simulink model "ADU_Integration_Y2016_simulation"  (R2016b)
settings: Solver=FixedStepDiscrete  StartTime=240  StopTime=300  FixedStep=0.01  RelTol=1e-3  EnableMultiTasking=on
PostLoadFcn:
  | , if any(exist('dsrtsu_mdlpostloadfcn', 'file') == [2, 3, 6]), try dsrtsu_mdlpostloadfcn('Execute', bdroot); catch fprintf('Error in PostLoadFcn (dsrtsu_mdlpostloadfcn) for model "%s":\n %s\n', bdroot, lasterr); end, end,
InitFcn:
  | load 'data/chi2_dat';
  | load 'data/innerLine_struct';
  | load 'data/middleLine_struct';
  | load 'data/outerLine_struct';
  | load 'data/innerLine';
  | load 'data/middleLine';
  | load 'data/outerLine';
  | load 'data/landmarks_patac_schimmel_ccw';
  | load 'data/patac_navi_array';
  | load 'data/sensor';
  | load 'data/map_struct';
  | addpath map_src
  | Integration_Parameter;
  | load 'TestData_001';
values from neighbouring files (symbols this model uses):
  TestData_001 =     [TestData_001.mat]
undefined symbols (not defined in the file or in its folder): chi2_dat, innerLine, landmarks_patac_schimmel_ccw, middleLine, outerLine, patac_navi_array
libraries: simulink x36, rtican x1
(part 1 of 20)
settings Model: DSRTSU_INTERNAL_RTI_VER=460  DSRTSU_INTERNAL_RTI_TYPE=rti1401  DSRTSU_INTERNAL_RTIFLEXRAYCONFIG=10  DSRTSU_INTERNAL_RTIFPGA=50  Creator=si8cwy  LastModifiedBy=Administrator
settings DataIOCC: LimitDataPoints=on  SaveFormat=Array  SignalLoggingSaveFormat=ModelDataLogs
settings OptimizationCC: BlockReduction=off  ConditionallyExecuteInputs=off  OptimizeBlockIOStorage=off  BufferReuse=off  GlobalBufferReuse=off  ExpressionFolding=off  ExpressionDepthLimit=2147483647  LocalBlockOutputs=off  RollThreshold=100  LifeSpan=inf
settings DebuggingCC: SolverPrmCheckMsg=warning  MultiTaskDSMMsg=warning  MultiTaskCondExecSysMsg=none  StateNameClashWarn=warning  SFUnexpectedBacktrackingDiag=warning  SFNoUnconditionalDefaultTransitionDiag=warning  SFExecutionAtInitializationDiag=none
settings HardwareCC: ProdBitPerPointer=32  ProdBitPerSizeT=32  ProdBitPerPtrDiffT=32  ProdLargestAtomicFloat=None  ProdEndianess=BigEndian  ProdWordSize=32  ProdHWDeviceType=Generic->Custom  TargetIntDivRoundTo=Zero  TargetEndianess=BigEndian  TargetHWDeviceType=Generic->Custom
settings ModelReferenceCC: PropagateSignalLabelsOutOfModel=off
settings RTWCC: SystemTargetFile=rti1401.tlc  MakeCommand=make_rti  TemplateMakefile=rti1401.tmf  Description=dSPACE DS1401 Hardware Platform
settings STFCustomTargetCC: ParMdlRefBuildCompliant=on  SystemTargetFile=rti1401.tlc
settings GRTTargetCC: TargetLangStandard=C89/C90 (ANSI)  CompOptLevelCompliant=off  ConcurrentExecutionCompliant=off  CombineOutputUpdateFcns=off  MatFileLogging=off  CPPClassGenCompliant=off  GRTInterface=on  UseToolchainInfoCompliant=off  ExtModeMexFile=noextcomm
settings ConfigComp: CovMetricSettings=dw  CovHtmlReporting=on  CovSaveCumulativeToWorkspaceVar=on  CovSaveSingleToWorkspaceVar=on  CovExternalEMLEnable=off  CovSFcnEnable=off

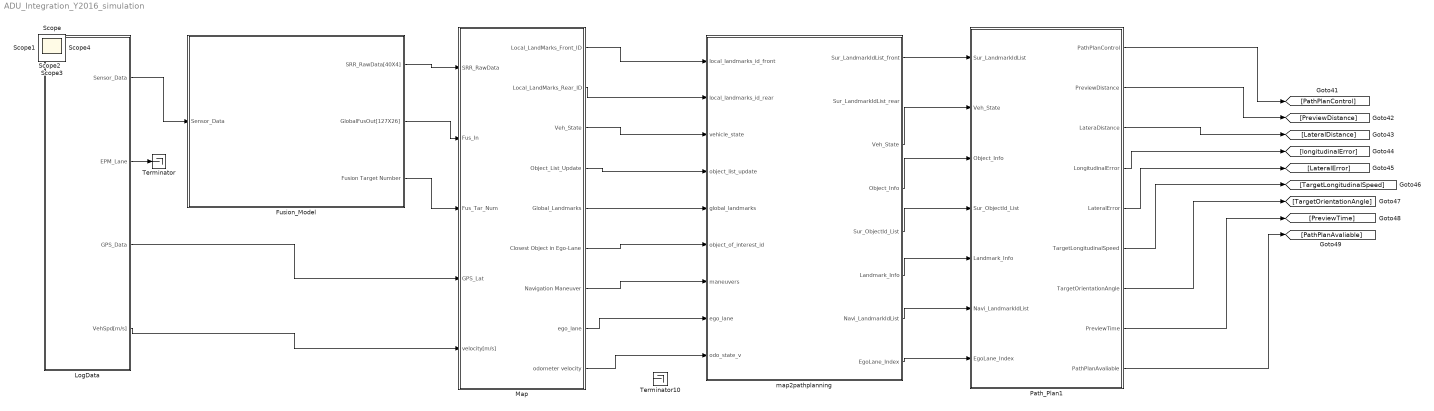
== system ADU_Integration_Y2016_simulation ==
  Fusion_Model : Subsystem
  LogData : Subsystem
  Map : Subsystem
  Path_Plan1 : Subsystem
  Terminator : Terminator
  Terminator10 : Terminator
  map2pathplanning : MATLAB Function  TreatAsAtomicUnit=on
  Scope{,1..4} (5 alike) : Scope
  wires:
  LogData/1(Sensor_Data) -> Fusion_Model/1(Sensor_Data)
  LogData/2(EPM_Lane) -> Terminator/1
  Path_Plan1/1(PathPlanControl) -> [PathPlanControl]
  Path_Plan1/2(PreviewDistance) -> [PreviewDistance]
  Path_Plan1/3(LateraDistance) -> [LateralDistance]
  Path_Plan1/9(PathPlanAvaliable) -> [PathPlanAvaliable]
  Path_Plan1/8(PreviewTime) -> [PreviewTime]
  Path_Plan1/4(LongitudinalError) -> [longitudinalError]
  Path_Plan1/5(LateralError) -> [LateralError]
  Path_Plan1/7(TargetOrientationAngle) -> [TargetOrientationAngle]
  Path_Plan1/6(TargetLongitudinalSpeed) -> [TargetLongitudinalSpeed]
  map2pathplanning/8(EgoLane_Index) -> Path_Plan1/7(EgoLane_Index)
  map2pathplanning/7(Navi_LandmarkIdList) -> Path_Plan1/6(Navi_LandmarkIdList)
  map2pathplanning/5(Sur_ObjectId_List) -> Path_Plan1/4(Sur_ObjectId_List)
  map2pathplanning/3(Veh_State) -> Path_Plan1/2(Veh_State)
  map2pathplanning/4(Object_Info) -> Path_Plan1/3(Object_Info)
  map2pathplanning/1(Sur_LandmarkIdList_front) -> Path_Plan1/1(Sur_LandmarkIdList)
  map2pathplanning/6(Landmark_Info) -> Path_Plan1/5(Landmark_Info)
  Map/1(Local_LandMarks_Front_ID) -> map2pathplanning/1(local_landmarks_id_front)
  Map/3(Veh_State) -> map2pathplanning/3(vehicle_state)
  Map/4(Object_List_Update) -> map2pathplanning/4(object_list_update)
  Map/5("Global_Landmarks ") -> map2pathplanning/5(global_landmarks)
  Map/6(Closest Object in Ego-Lane) -> map2pathplanning/6(object_of_interest_id)
  Map/7(Navigation Maneuver) -> map2pathplanning/7(maneuvers)
  Map/9(odometer velocity) -> map2pathplanning/9(odo_state_v)
  Map/8(ego_lane) -> map2pathplanning/8(ego_lane)
  Fusion_Model/2(GlobalFusOut[127X26]) -> Map/2(Fus_In)
  Fusion_Model/1(SRR_RawData[40X4]) -> Map/1(SRR_RawData)
  LogData/3(GPS_Data) -> Map/4(GPS_Lat)
  LogData/4(VehSpd[m/s]) -> Map/5(velocity[m/s])
  Map/2(Local_LandMarks_Rear_ID) -> map2pathplanning/2(local_landmarks_id_rear)
  Fusion_Model/3(Fusion Target Number) -> Map/3(Fus_Tar_Num)

== system ADU_Integration_Y2016_simulation/Fusion_Model ==
  note: SRR  Data
      | --------------------------------------------------------
      | |  1  |     2       |      3       |       4       |
      | --------------------------------------------------------
      | | ID | RangeX | RangeY | MoveInfo |
  note: Model Description:
      | This Model now don't take SRR Data to initial fusion tracker, the side fusion strategy will develop and update the model,
      | all output is based on vehicle coordinate, which original point located on the front middle of vehicle, the vehicle is 1.8m
      | wide and 5.2m long. Now the Move Info signal and Fus_State is unavialbe, The fusion output has two way, the 127x26
      | and 127 object is optional,the EPM Obstacle is used for ACC Strategy, not used for path plan and motion control.
  note: FusDataOut  Data
      | ------------------------------------------------------------------------------------------------------------------------------------------------------------------------------------------------------------------------------------------------------------------------------------------------------
      | |  1  |     2       |   3    |     4        |    5   |        6       |   7      |   8    |        9        |         10      |   11  |  12  |  13  |  14   | 15   |  16  |  17   |  18  |  19  |   20  |  21  |  22  |   23  |  24  |  25  |  26   |
      | -----------------------------------------------------------------------------------------------------------------------------------------------------------------------------------------------------------------------------------------------------------------------------------------------------
      | | ID | RangeX | VelX | RangeY | VelY | MoveInfo | Width | Type | Fus_State | Confidence| P11 | P12 | P13 | P14 | P21 | P22 | P23 | P24 | P31 | P32 | P33 | P34 | P41 | P42 | P43 | P44 |
  Sensor_Data : Inport
  DocBlock : simulink/Model-Wide Utilities/DocBlock  DocumentType=Text
      content=|
      | V1.0
      | 2016/11/1   |   First Release
      | V2.0
      | 2016/11/7   |   Changelog:
      | 1)  Output all SRR Raw Data, used for map;
      | 2)  Updating EPM dbc, new feature is avaliable;
      | 3)  Add Obstacle_State A/B/C for acc control;
      | 4)  Add FreeSpace and HPP signal for other use.
  Fusion_Block : Subsystem
  To Workspace : ToWorkspace  VariableName=FusOut  SampleTime=-1
  SRR_RawData[40X4] : Outport
  GlobalFusOut[127X26] : Outport  Port=2
  Fusion Target Number : Outport  Port=3
  wires:
  Fusion_Block/1(Fus_Data_Out) -> To Workspace/1, GlobalFusOut[127X26]/1
  Fusion_Block/3(SRR_RawData) -> SRR_RawData[40X4]/1
  Sensor_Data/1 -> Fusion_Block/1(Sensor_Data)
  Fusion_Block/2(fusion target number) -> Fusion Target Number/1

== system ADU_Integration_Y2016_simulation/LogData ==
  1-D Lookup Table2 : Lookup_n-D  NumberOfTableDimensions=1  BreakpointsForDimension1=TestData_001.X.Data  Table=TestData_001.Y(731).Data  RndMeth=Simplest  InputSameDT=on
  Bus Creator : BusCreator  Inputs=6
  Clock : Clock
  LF_SRR_Data : Subsystem
  LR_SRR_Data : Subsystem
  RF_SRR_Data : Subsystem
  RR_SRR_Data : Subsystem
  SER_M2S : Subsystem
  Sensor_ESR : Subsystem
  Vision_Target : Subsystem
  Sensor_Data : Outport
  EPM_Lane : Outport  Port=2
  GPS_Data : Outport  Port=3
  VehSpd[m/s] : Outport  Port=4
  tag scope: Clock=global
  wires:
  LF_SRR_Data/1(LF_SRR_Data[10x5]) -> Bus Creator/2  "LF_SRR_Data[10X5]"
  RF_SRR_Data/1(RF_SRR_Data[10x5]) -> Bus Creator/3  "RF_SRR_Data[10X5]"
  LR_SRR_Data/1(LR_SRR_Data[10x5]) -> Bus Creator/4  "LR_SRR_Data[10X5]"
  RR_SRR_Data/1(RR_SRR_Data[10x5]) -> Bus Creator/5  "RR_SRR_Data[10X5]"
  Vision_Target/1(Vision_Target[25x8]) -> Bus Creator/6  "Vision_Target[25X8]"
  Bus Creator/1 -> Sensor_Data/1  "Sensor_Veh_Data"
  Sensor_ESR/1(ESR_Data[64X4]) -> Bus Creator/1  "ESR_Data[64X4]"
  Vision_Target/2(EPM_Lane) -> EPM_Lane/1
  Clock/1 -> [Clock]
  SER_M2S/1(NET_Output) -> GPS_Data/1
  [Clock] -> 1-D Lookup Table2/1
  1-D Lookup Table2/1 -> VehSpd[m/s]/1

== system ADU_Integration_Y2016_simulation/Map ==
  SRR_RawData : Inport
  Fus_In : Inport  Port=2
  Fus_Tar_Num : Inport  Port=3
  GPS_Lat : Inport  Port=4
  velocity[m/s] : Inport  Port=5
  Bus Selector2 : BusSelector  OutputSignals=GPGLL.Y_Lat,GPGLL.Y_Long,GPHPR.Crouse_Range,GPGLL.Time[s]
  Constant : Constant  Value=chi2_dat
  Constant1 : Constant  Value=middleLine  OutDataTypeStr=Bus: middleLine_struct
  Constant2 : Constant  Value=innerLine  OutDataTypeStr=Bus: innerLine_struct
  Constant3 : Constant  Value=outerLine  OutDataTypeStr=Bus: outerLine_struct
  Constant5 : Constant  Value=patac_navi_array  OutDataTypeStr=double
  Data Store Memory2 : DataStoreMemory  DataStoreName=chi2  ReadBeforeWriteMsg=warning  WriteAfterWriteMsg=warning  WriteAfterReadMsg=warning  InitialValue=zeros(1,1000)  ShowAdditionalParam=off  OutDataTypeStr=double
  Display : Display
  Map_Navigation : MATLAB Function  TreatAsAtomicUnit=on
  Terminator4 : Terminator
  landmarks_patac_schimmel_ccw : Constant  Value=landmarks_patac_schimmel_ccw  OutDataTypeStr=double
  Local_LandMarks_Front_ID : Outport
  Local_LandMarks_Rear_ID : Outport  Port=2
  Veh_State : Outport  Port=3
  Object_List_Update : Outport  Port=4
  "Global_Landmarks " : Outport  Port=5
  Closest Object in Ego-Lane : Outport  Port=6
  Navigation Maneuver : Outport  Port=7
  ego_lane : Outport  Port=8
  odometer velocity : Outport  Port=9
  wires:
  Map_Navigation/3(object_list_update) -> Object_List_Update/1
  Map_Navigation/2(vehicle_state) -> Display/1, Veh_State/1
  velocity[m/s]/1 -> Map_Navigation/6(odo_motion_v)
  GPS_Lat/1 -> Bus Selector2/1
  Bus Selector2/1 -> Map_Navigation/7(rtk_gps_lat)  "<Y_Lat>"
  Bus Selector2/2 -> Map_Navigation/8(rtk_gps_lon)  "<Y_Long>"
  Bus Selector2/3 -> Map_Navigation/9(rtk_gps_yaw)  "<Crouse_Range>"
  Bus Selector2/4 -> Map_Navigation/10(rtk_gps_ts)  "<Time[s]>"
  SRR_RawData/1 -> Map_Navigation/11(sensor_data_raw)
  Fus_In/1 -> Map_Navigation/12(object_list)
  Map_Navigation/4(object_of_interest_id) -> Closest Object in Ego-Lane/1
  Map_Navigation/7(maneuvers) -> Navigation Maneuver/1
  Constant/1 -> Map_Navigation/1(chi2_dat)
  Constant2/1 -> Map_Navigation/2(innerLine)
  Constant1/1 -> Map_Navigation/3(middleLine)
  Constant3/1 -> Map_Navigation/4(outerLine)
  landmarks_patac_schimmel_ccw/1 -> Map_Navigation/5(landmarks)
  Constant5/1 -> Map_Navigation/14(patac_navi)
  ? -> Terminator4/1
  Map_Navigation/12(odo_state_v) -> odometer velocity/1
  Map_Navigation/5(landmarks_in_proximity_id_in_front) -> Local_LandMarks_Front_ID/1
  Map_Navigation/1(global_landmarks) -> "Global_Landmarks "/1
  Map_Navigation/11(ego_location) -> ego_lane/1
  Map_Navigation/6(landmarks_in_proximity_id_in_rear) -> Local_LandMarks_Rear_ID/1
  Fus_Tar_Num/1 -> Map_Navigation/13(object_num)

== system ADU_Integration_Y2016_simulation/Path_Plan1 ==
  note: Veh_State
      | |  1 |  2  |    3   |  4  |  5  |  6  |  7  | 8 |
      | -------------------------------------------------
      | | X  | Y  | Beta | Vx | Vy | Ax | Ay | V |
  note: FusDataOut  Data
      | ------------------------------------------------------------------------------------------------------------------------------------------------------------------------------------------------------------------------------------------------------
      | |  1  |     2       |   3    |     4        |    5   |        6       |   7      |   8    |        9        |         10      |   11  |  12  |  13  |  14   | 15   |  16  |  17   |  18  |  19  |   20  |  21  |  22  |   23  |  24  |  25  |  26   |
      | -------------------------------------------------------------------------------------------------------------------------------------------------------------------------------------------------------------------------------------------------------
      | | ID | RangeX | VelX | RangeY | VelY | MoveInfo | Width | Type | Fus_State | Confidence| P11 | P12 | P13 | P14 | P21 | P22 | P23 | P24 | P31 | P32 | P33 | P34 | P41 | P42 | P43 | P44 |
  note: Landmark_Info
      | |   1  |   2   |   3   |   4  |    5    |
      | ---------------------------------------- X 30
      | | X1  | Y1  |  X2  |  Y2 | Type |
  note: Sur_LandmarkIdList
      | |  1  |  2  |  3  |  4  |  5  |  6  |  7  |  8  |  9  |  10  |
      | --------------------------------------------------------------
      | | id  |
  note: Navi_LandmarkIdList
      | |  1  |  2  |      3      |    4   |
      | ----------------------------------
      | |  x  |  y  |  Range  |  OP  |
  note: Sur_ObjectId_List
      | |  1  |  2  |  3  |  4  |
      | -------------------------  1stLane   2ndLane  3rdLane
      | | id  |
  Sur_LandmarkIdList : Inport
  Veh_State : Inport  Port=2
  Object_Info : Inport  Port=3
  Sur_ObjectId_List : Inport  Port=4
  Landmark_Info : Inport  Port=5
  Navi_LandmarkIdList : Inport  Port=6
  EgoLane_Index : Inport  Port=7
  Constant : Constant
  CordTransfer : MATLAB Function  TreatAsAtomicUnit=on
  CordTransfer1 : MATLAB Function  TreatAsAtomicUnit=on
  Demux : Demux
  Demux1 : Demux
  Demux2 : Demux  Outputs=8
  InterSectionPathPlanningModule : Subsystem
  LaneChangePathPlanningModule1 : Subsystem
  PathArbModule : Subsystem
  SceneSelectionModule : Subsystem
  Terminator : Terminator
  Terminator1 : Terminator
  Terminator2 : Terminator
  Unit Delay : UnitDelay  InitialCondition=1  SampleTime=-1
  PathPlanControl : Outport
  PreviewDistance : Outport  Port=2
  LateraDistance : Outport  Port=3
  LongitudinalError : Outport  Port=4
  LateralError : Outport  Port=5
  TargetLongitudinalSpeed : Outport  Port=6
  TargetOrientationAngle : Outport  Port=7
  PreviewTime : Outport  Port=8
  PathPlanAvaliable : Outport  Port=9
  wires:
  Unit Delay/1 -> SceneSelectionModule/8(OperationFinishFlg)
  PathArbModule/6(PathTrigFinishFlg) -> Unit Delay/1
  LaneChangePathPlanningModule1/6(PathTrigFinishFlg) -> PathArbModule/12(PathTrigFinishFlgLC)
  InterSectionPathPlanningModule/6(PathTrigFinishFlg) -> PathArbModule/6(PathTrigFinishFlgInter)
  LaneChangePathPlanningModule1/5(PreViewTime) -> PathArbModule/11(PreviewTimeLC)
  LaneChangePathPlanningModule1/4(TargetThetalo) -> PathArbModule/10(TargetThetaLoLC)
  LaneChangePathPlanningModule1/3(PathPlanningSuccessFlg) -> PathArbModule/9(VePathPlan_e_LCPPSucFlg)
  LaneChangePathPlanningModule1/2(VsPathPlan_h_Motion) -> PathArbModule/8(VsPathPlan_h_LCMotion)
  LaneChangePathPlanningModule1/1(VsPathPlan_h_position) -> PathArbModule/7(VsPathPlan_h_LCposition)
  InterSectionPathPlanningModule/5(PreViewTime) -> PathArbModule/5(PreviewTimeInter)
  InterSectionPathPlanningModule/4(TargetThetalo) -> PathArbModule/4(TargetThetaLoInter)
  InterSectionPathPlanningModule/3(PathPlanningSuccessFlg) -> PathArbModule/3(VePathPlan_e_InterPPSucFlg)
  InterSectionPathPlanningModule/2(VsPathPlan_h_Motion) -> PathArbModule/2(VsPathPlan_h_InterSecMotion)
  InterSectionPathPlanningModule/1(VsPathPlan_h_position) -> PathArbModule/1(VsPathPlan_h_InterSecposition)
  PathArbModule/3(VePathPlan_b_InChargFlg) -> PathPlanControl/1
  PathArbModule/2(VsPathPlan_h_Motion) -> Demux1/1, CordTransfer1/3(VsPathPlan_h_MotionPGC)
  PathArbModule/1(VsPathPlan_h_position) -> Demux/1, CordTransfer1/2(VsPathPlan_h_positionPGC)
  PathArbModule/5(PreviewTime) -> PreviewTime/1
  PathArbModule/4(TargetThetaLo) -> TargetOrientationAngle/1, CordTransfer1/4(TargetThetaLoPGC)
  Demux1/1 -> TargetLongitudinalSpeed/1
  Demux/4 -> LateralError/1
  Demux/3 -> LongitudinalError/1
  Demux/2 -> LateraDistance/1
  Demux/1 -> PreviewDistance/1
  Constant/1 -> PathPlanAvaliable/1
  CordTransfer/6(Info_LoPGCd) -> LaneChangePathPlanningModule1/10(Info_Lo)
  CordTransfer/5(Info_LdPGCd) -> InterSectionPathPlanningModule/4(Info_Ld), LaneChangePathPlanningModule1/9(Info_Ld)
  CordTransfer/3(Info_FdPGCd) -> InterSectionPathPlanningModule/5(Info_Fd), LaneChangePathPlanningModule1/7(Info_Fd)
  Demux2/2 -> InterSectionPathPlanningModule/7(YposLoCur), LaneChangePathPlanningModule1/3(YposLoCur)
  Demux2/3 -> InterSectionPathPlanningModule/8(ThetaLoCur), LaneChangePathPlanningModule1/4(ThetaLoCur)
  CordTransfer/4(Info_FoPGCd) -> LaneChangePathPlanningModule1/8(Info_Fo)
  CordTransfer/1(Info_MePGCd) -> InterSectionPathPlanningModule/1(Info_Me), LaneChangePathPlanningModule1/1(Info_Me)
  Demux2/1 -> InterSectionPathPlanningModule/6(XposLoCur), LaneChangePathPlanningModule1/2(XposLoCur)
  CordTransfer/8(CurOpPGCd) -> InterSectionPathPlanningModule/3(VePathPlanning_e_CurOp), LaneChangePathPlanningModule1/6(VePathPlanning_e_CurOp), PathArbModule/13(VePathPlan_e_OutputSelection)
  Sur_LandmarkIdList/1 -> SceneSelectionModule/1(Sur_LandmarkIdList)
  Veh_State/1 -> Demux2/1, SceneSelectionModule/2(Veh_State)
  Navi_LandmarkIdList/1 -> SceneSelectionModule/6(Navi_LandmarkIdList)
  Landmark_Info/1 -> SceneSelectionModule/5(Landmark_Info)
  Sur_ObjectId_List/1 -> SceneSelectionModule/4(Sur_ObjectId_List)
  Object_Info/1 -> SceneSelectionModule/3(Object_Info)
  EgoLane_Index/1 -> SceneSelectionModule/7(EgoLane_Index)
  CordTransfer/2(RoadInfoPGCd) -> InterSectionPathPlanningModule/2(RoadInfo), LaneChangePathPlanningModule1/5(RoadInfo)
  CordTransfer/7(LongDisLimitPGCd) -> LaneChangePathPlanningModule1/11(LongDisLimit)
  SceneSelectionModule/1(Info_Me) -> CordTransfer/1(Info_MeGCd)
  SceneSelectionModule/2(Info_Fd) -> CordTransfer/2(Info_FdGCd)
  SceneSelectionModule/3(Info_Fo) -> CordTransfer/3(Info_FoGCd)
  SceneSelectionModule/5(Info_Lo) -> CordTransfer/5(Info_LoGCd)
  SceneSelectionModule/6(CurOp) -> CordTransfer/6(CurOpGCd)
  SceneSelectionModule/4(Info_Ld) -> CordTransfer/4(Info_LdGCd)
  SceneSelectionModule/7(LongDisLimit) -> CordTransfer/7(LongDisLimitGCd)
  SceneSelectionModule/8(RoadInfo) -> CordTransfer/8(RoadInfoGCd)
  CordTransfer/9(PGCdInfo) -> CordTransfer1/1(PGCdInfo)
  CordTransfer1/3(TargetThetaLo) -> Terminator2/1
  CordTransfer1/2(VsPathPlan_h_Motion) -> Terminator1/1
  CordTransfer1/1(VsPathPlan_h_position) -> Terminator/1

== system ADU_Integration_Y2016_simulation/Fusion_Model/Fusion_Block ==
  Sensor_Data : Inport
  Bus Selector : BusSelector  OutputSignals=Total_Targ_Num
  Display : Display
  Fus_Header_Gen : Subsystem
  Global_Fusion : Subsystem
  Side_Fusion : Subsystem
  Terminator : Terminator
  Fus_Data_Out : Outport
  fusion target number : Outport  Port=2
  SRR_RawData : Outport  Port=3
  wires:
  Side_Fusion/1(SideFus_Output[40X4]) -> Global_Fusion/1(From SideFusion)
  Global_Fusion/1(GlobalFusOut[127X26]) -> Fus_Data_Out/1
  Sensor_Data/1 -> Side_Fusion/1(From Sensor), Global_Fusion/2(From Sensor)
  Global_Fusion/2(Total_TargetNum) -> Display/1, Fus_Header_Gen/1(Target_Num)
  Side_Fusion/2(SideRadar_RawData[40X4]) -> SRR_RawData/1
  Fus_Header_Gen/1(Fus_Header) -> Bus Selector/1, Terminator/1
  Bus Selector/1 -> fusion target number/1  "<Total_Targ_Num>"

== system ADU_Integration_Y2016_simulation/LogData/LF_SRR_Data ==
  note: This part is used for ensure the sensor data is from once update
  1-D Lookup Table : Lookup_n-D  NumberOfTableDimensions=1  BreakpointsForDimension1=TestData_001.X.Data  Table=TestData_001.Y(51).Data  RndMeth=Simplest  InputSameDT=on
  Chart : Stateflow chart  TreatAsAtomicUnit=on
  LFSRR_Data : Subsystem
  LF_SRR_Data[10x5] : Outport
  tag scope: LFSRRTime=global, LFSRRcal=global
  wires:
  LFSRR_Data/1(LFSRR[10X5]) -> Chart/2(DataInput)
  1-D Lookup Table/1 -> Chart/1(Trig), [LFSRRcal]
  Chart/1(DataOutput) -> LF_SRR_Data[10x5]/1
  [Clock] -> Chart/3(Time), 1-D Lookup Table/1
  Chart/2(Time_out) -> [LFSRRTime]

== system ADU_Integration_Y2016_simulation/LogData/LR_SRR_Data ==
  1-D Lookup Table : Lookup_n-D  NumberOfTableDimensions=1  BreakpointsForDimension1=TestData_001.X.Data  Table=TestData_001.Y(51*2).Data  RndMeth=Simplest  InputSameDT=on
  Chart : Stateflow chart  TreatAsAtomicUnit=on
  LRSRR_Data : Subsystem  mask{StartNum=52}
  Rate Transition3 : RateTransition  Deterministic=off
  LR_SRR_Data[10x5] : Outport
  tag scope: LRSRRTime=global, LRSRRcal=global
  wires:
  Chart/1(DataOutput) -> Rate Transition3/1
  1-D Lookup Table/1 -> Chart/1(Trig), [LRSRRcal]
  Rate Transition3/1 -> LR_SRR_Data[10x5]/1
  [Clock] -> Chart/3(Time), 1-D Lookup Table/1
  LRSRR_Data/1(LRSRR[10X5]) -> Chart/2(DataInput)
  Chart/2(Time_out) -> [LRSRRTime]

== system ADU_Integration_Y2016_simulation/LogData/RF_SRR_Data ==
  1-D Lookup Table : Lookup_n-D  NumberOfTableDimensions=1  BreakpointsForDimension1=TestData_001.X.Data  Table=TestData_001.Y(153).Data  RndMeth=Simplest  InputSameDT=on
  Chart : Stateflow chart  TreatAsAtomicUnit=on
  RFSRR_Data : Subsystem  mask{StartNum=103}
  RF_SRR_Data[10x5] : Outport
  tag scope: RFSRRTime=global, RFSRRcal=global
  wires:
  1-D Lookup Table/1 -> Chart/1(Trig), [RFSRRcal]
  Chart/1(DataOutput) -> RF_SRR_Data[10x5]/1
  [Clock] -> Chart/3(Time), 1-D Lookup Table/1
  RFSRR_Data/1(RFSRR[10X5]) -> Chart/2(DataInput)
  Chart/2(Time_out) -> [RFSRRTime]

== system ADU_Integration_Y2016_simulation/LogData/RR_SRR_Data ==
  1-D Lookup Table : Lookup_n-D  NumberOfTableDimensions=1  BreakpointsForDimension1=TestData_001.X.Data  Table=TestData_001.Y(51*4).Data  RndMeth=Simplest  InputSameDT=on
  Chart : Stateflow chart  TreatAsAtomicUnit=on
  LRSRR_Data : Subsystem  mask{StartNum=154}
  RR_SRR_Data[10x5] : Outport
  tag scope: RRSRRTime=global, RRSRRcal=global
  wires:
  LRSRR_Data/1(RRSRR[10X5]) -> Chart/2(DataInput)
  [Clock] -> Chart/3(Time), 1-D Lookup Table/1
  1-D Lookup Table/1 -> Chart/1(Trig), [RRSRRcal]
  Chart/1(DataOutput) -> RR_SRR_Data[10x5]/1
  Chart/2(Time_out) -> [RRSRRTime]

== system ADU_Integration_Y2016_simulation/LogData/SER_M2S ==
  1-D Lookup Table1 : Lookup_n-D  NumberOfTableDimensions=1  BreakpointsForDimension1=TestData_001.X.Data  Table=TestData_001.Y(739).Data  RndMeth=Simplest  InputSameDT=on
  1-D Lookup Table2 : Lookup_n-D  NumberOfTableDimensions=1  BreakpointsForDimension1=TestData_001.X.Data  Table=TestData_001.Y(738).Data  RndMeth=Simplest  InputSameDT=on
  1-D Lookup Table3 : Lookup_n-D  NumberOfTableDimensions=1  BreakpointsForDimension1=TestData_001.X.Data  Table=TestData_001.Y(740).Data  RndMeth=Simplest  InputSameDT=on
  1-D Lookup Table4 : Lookup_n-D  NumberOfTableDimensions=1  BreakpointsForDimension1=TestData_001.X.Data  Table=TestData_001.Y(740).Data  RndMeth=Simplest  InputSameDT=on
  1-D Lookup Table5 : Lookup_n-D  NumberOfTableDimensions=1  BreakpointsForDimension1=TestData_001.X.Data  Table=TestData_001.Y(734).Data  RndMeth=Simplest  InputSameDT=on
  1-D Lookup Table6 : Lookup_n-D  NumberOfTableDimensions=1  BreakpointsForDimension1=TestData_001.X.Data  Table=TestData_001.Y(735).Data  RndMeth=Simplest  InputSameDT=on
  1-D Lookup Table7 : Lookup_n-D  NumberOfTableDimensions=1  BreakpointsForDimension1=TestData_001.X.Data  Table=TestData_001.Y(736).Data  RndMeth=Simplest  InputSameDT=on
  Bus Creator : BusCreator  Inputs=3
  Bus Creator1 : BusCreator  Inputs=4
  Bus Creator2 : BusCreator  Inputs=2
  NET_Output : Outport
  wires:
  1-D Lookup Table3/1 -> Bus Creator/3  "Time[s]"
  1-D Lookup Table2/1 -> Bus Creator/1  "Y_Lat"
  1-D Lookup Table1/1 -> Bus Creator/2  "Y_Long"
  Bus Creator2/1 -> NET_Output/1
  Bus Creator1/1 -> Bus Creator2/2  "GPHPR"
  1-D Lookup Table6/1 -> Bus Creator1/3  "Pitch_angle"
  1-D Lookup Table5/1 -> Bus Creator1/2  "Crouse_Range"
  Bus Creator/1 -> Bus Creator2/1  "GPGLL"
  1-D Lookup Table4/1 -> Bus Creator1/1  "Time"
  1-D Lookup Table7/1 -> Bus Creator1/4  "Roll_angle"
  [Clock] -> 1-D Lookup Table2/1, 1-D Lookup Table1/1, 1-D Lookup Table7/1, 1-D Lookup Table6/1, 1-D Lookup Table5/1, 1-D Lookup Table4/1, 1-D Lookup Table3/1

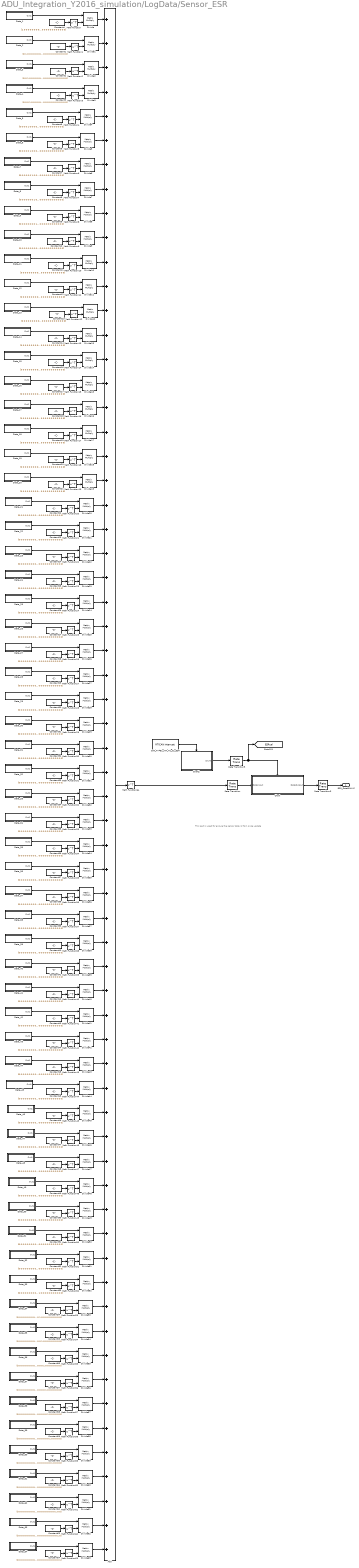
== system ADU_Integration_Y2016_simulation/LogData/Sensor_ESR ==
  note: This part is used for ensure the sensor data is from once update
  Add : Sum  Inputs=++++++++++++++++++++++++++++++++++++++++++++++++++++++++++++++++
  CAN_TYPE1_INT_M1_C1_ESR : rtican/RTICAN Interrupt  Reserved1=[]  Reserved2=[]  Reserved3=[]  Reserved4=[]  BoardTypeNo=[]  BoardNo=[]  ChannelNo=[]  Parameters=[]  InterruptName=[]  BoardIntNo=[]  Sfcn_Int_Struct=[]  BoardType=[]  SintNo=[]  Int_Struct=[]  DialogFcn=[]  UnitName=[]  Revision=[]  UnitValues=[]  DSProperties=struct('RTI',struct('Version',uint32(4),'BlockType',struct('isSLSource',uint8(1),'isSLSink',uint8(0),'isHWSource',uint8(1),'isHWSink',uint8(0),'isSetup',uint8(0),'isInline',uint8(1),'isNonInline',uint8(0),'isInterrupt',uint8(1),'isChannelwise',uint8(0)),'IOBoardType','RTICAN','UnitType','HWINT','Identifier','CANINT','DialogType','ML','BlockSet','RTICAN','RelationId',struct('TH',struct('BlockId','HWINT')),'SlaveProcessor','CAN'))  RTIBlockInterface=struct('OutputPortsWidth',int32(1),'FunctionCall',uint32(0),'OutputPortsActive',1,'DialogFcn','rtican_interrupt_gui','BlockDisplay',{{['CAN RX Interrupt'],'center'}},'IconTransparency','off','ParameterTunableNames',{{}},'InitLevel',3,'BlockName',struct('Token',{{'CAN_TYPE','_INT_M','_C'}},'BlockParam',{{'BoardTypeNo','BoardNo','ChannelNo'}}),'Options',{{'SS_OPTION_FORCE_NONINLINED_FCNCALL','SS_OPTION_ASYNCHRONOUS_INTERRUPT'}})  RTIBlockParameters=struct('BoardTypeNo',{{1,'OFF',[]}},'BoardNo',{{2,'ON',[1 16]}},'ChannelNo',{{2,'ON',[1 2]}},'Parameters',{{struct('general',struct('Type','RX','NumFormat','hex','MsgIdFormat','STD','MsgId',1343,'isFromLib',0)),'OFF',[]}},'GroupId',{{struct('Group','RTICAN','No',2,'Behavior','NAMECHANGE','BlockType','SINK','NameChangeFlag',0),'OFF',[]}},'SFcnRTICANInterrupt',{{0,'OFF',[]}},'ThSrcSgnName',{{['CAN_TYPE1_M2_C2 RX Interrupt'],'OFF',[]}},'ThBlk',{{['struct(''blkh'',''ADU_Integration_Y2016_simulation/LogData/Sensor_ESR/CAN_TYPE1_INT_M1_C1_ESR'',''srcId'',''CAN6'',''srcSgnId'',''CAN6'',''intervalTmrBlockId'',[],''srcSgnName'',[''CAN_TYPE1_M2_C2 RX Interrupt''],''srcCpuId'','''',''isSrcCpu'',1,''isTargetCpu'',1,''srcOnMasterCpu'',1,''boardType'',''CAN'',''boardTypeNo'',''1'',''boardNo'',1,''intNo'',2,''subIntNo'',-1,''period'',0,''entryPoint'',''rti_CAN6'',''blockName'',''CAN_TYPE1_INT_M1_C1_ESR'',''taskNameDisplayExt'','''',''taskType'',''HWINT'',''groupId'',''CANINT1B2'',''hookFcn'',''NULL'',''isTimerTaskSrc'',0,''service'','''',''mpBlkId'','''',''taskPriorityPreConfig'',''none'',''taskPriority'',-1,''taskSortWeighting'',[],''taskSchedulingPolicy'',''FCFS'',''taskOvrPreConfig'',''none'',''taskOvrStrategy'',1,''taskOvrQueueSize'',1,''taskVisibility'',''on'',''taskGroupId'','''',''taskGroupDisplayOrder'',[],''serviceDynamicGen'',0,''disableCodeGen'',0,''boardBase'',''0'',''noBoardBase'','''')'],'OFF',[]}},'PHSBoardBaseId',{{'DS4302','OFF',[]}},'TLCFileName',{{'rtican_interrupt','OFF',[]}})  RTISFcnParameters=struct('SFcnRTICANInterrupt','struct','ThBlk','struct','PHSBoardBaseId','char','TLCFileName','char')  RTIBlockParaDefault=struct('BoardTypeNo',4302,'BoardNo',1,'ChannelNo',1,'Parameters',struct('general',struct('Type','RX','NumFormat','dec','MsgIdFormat','STD','MsgId',100,'isFromLib',1)),'GroupId',struct('Group',{{'RTICAN'}},'No',1,'Behavior',{{'NAMECHANGE'}},'BlockType',{{'SINK'}},'NameChangeFlag',0),'SFcnRTICANInterrupt',0,'ThSrcSgnName',['DS4302CAN_B1_C1 RX Interrupt'],'ThBlk',['struct(''srcSgnId'', '''')'],'PHSBoardBaseId','DS4302','TLCFileName','rtican_interrupt')
      settings: AttributesFormatString=Group Id: RTICAN2\n
  Chart : Stateflow chart  TreatAsAtomicUnit=on
  Chart2 : Stateflow chart  TreatAsAtomicUnit=on
  Constant1 : Constant  Value=[0 1 0 0 0 0 0 0 0 0 0 0 0 0 0 0 0 0 0 0 0 0 0 0 0 0 0 0 0 0 0 0 0 0 0 0 0 0 0 0 0 0 0 0 0 0 0 0 0 0 0 0 0 0 0 0 0 0 0 0 0 0 0 0]
  Constant10 : Constant  Value=[0 0 0 0 0 0 0 0 0 1 0 0 0 0 0 0 0 0 0 0 0 0 0 0 0 0 0 0 0 0 0 0 0 0 0 0 0 0 0 0 0 0 0 0 0 0 0 0 0 0 0 0 0 0 0 0 0 0 0 0 0 0 0 0]
  Constant11 : Constant  Value=[0 0 0 0 0 0 0 0 0 0 1 0 0 0 0 0 0 0 0 0 0 0 0 0 0 0 0 0 0 0 0 0 0 0 0 0 0 0 0 0 0 0 0 0 0 0 0 0 0 0 0 0 0 0 0 0 0 0 0 0 0 0 0 0]
  Constant12 : Constant  Value=[0 0 0 0 0 0 0 0 0 0 0 1 0 0 0 0 0 0 0 0 0 0 0 0 0 0 0 0 0 0 0 0 0 0 0 0 0 0 0 0 0 0 0 0 0 0 0 0 0 0 0 0 0 0 0 0 0 0 0 0 0 0 0 0]
  Constant13 : Constant  Value=[0 0 0 0 0 0 0 0 0 0 0 0 1 0 0 0 0 0 0 0 0 0 0 0 0 0 0 0 0 0 0 0 0 0 0 0 0 0 0 0 0 0 0 0 0 0 0 0 0 0 0 0 0 0 0 0 0 0 0 0 0 0 0 0]
  Constant14 : Constant  Value=[0 0 0 0 0 0 0 0 0 0 0 0 0 1 0 0 0 0 0 0 0 0 0 0 0 0 0 0 0 0 0 0 0 0 0 0 0 0 0 0 0 0 0 0 0 0 0 0 0 0 0 0 0 0 0 0 0 0 0 0 0 0 0 0]
  Constant15 : Constant  Value=[0 0 0 0 0 0 0 0 0 0 0 0 0 0 0 0 0 0 0 0 0 0 0 0 0 0 0 0 0 0 0 0 0 0 0 0 0 0 0 0 0 0 0 1 0 0 0 0 0 0 0 0 0 0 0 0 0 0 0 0 0 0 0 0]
  Constant16 : Constant  Value=[0 0 0 0 0 0 0 0 0 0 0 0 0 0 1 0 0 0 0 0 0 0 0 0 0 0 0 0 0 0 0 0 0 0 0 0 0 0 0 0 0 0 0 0 0 0 0 0 0 0 0 0 0 0 0 0 0 0 0 0 0 0 0 0]
  Constant17 : Constant  Value=[0 0 0 0 0 0 0 0 0 0 0 0 0 0 0 1 0 0 0 0 0 0 0 0 0 0 0 0 0 0 0 0 0 0 0 0 0 0 0 0 0 0 0 0 0 0 0 0 0 0 0 0 0 0 0 0 0 0 0 0 0 0 0 0]
  Constant18 : Constant  Value=[0 0 0 0 0 0 0 0 0 0 0 0 0 0 0 0 1 0 0 0 0 0 0 0 0 0 0 0 0 0 0 0 0 0 0 0 0 0 0 0 0 0 0 0 0 0 0 0 0 0 0 0 0 0 0 0 0 0 0 0 0 0 0 0]
  Constant19 : Constant  Value=[0 0 0 0 0 0 0 0 0 0 0 0 0 0 0 0 0 1 0 0 0 0 0 0 0 0 0 0 0 0 0 0 0 0 0 0 0 0 0 0 0 0 0 0 0 0 0 0 0 0 0 0 0 0 0 0 0 0 0 0 0 0 0 0]
  Constant2 : Constant  Value=[0 0 1 0 0 0 0 0 0 0 0 0 0 0 0 0 0 0 0 0 0 0 0 0 0 0 0 0 0 0 0 0 0 0 0 0 0 0 0 0 0 0 0 0 0 0 0 0 0 0 0 0 0 0 0 0 0 0 0 0 0 0 0 0]
  Constant20 : Constant  Value=[0 0 0 0 0 0 0 0 0 0 0 0 0 0 0 0 0 0 1 0 0 0 0 0 0 0 0 0 0 0 0 0 0 0 0 0 0 0 0 0 0 0 0 0 0 0 0 0 0 0 0 0 0 0 0 0 0 0 0 0 0 0 0 0]
  Constant21 : Constant  Value=[0 0 0 0 0 0 0 0 0 0 0 0 0 0 0 0 0 0 0 1 0 0 0 0 0 0 0 0 0 0 0 0 0 0 0 0 0 0 0 0 0 0 0 0 0 0 0 0 0 0 0 0 0 0 0 0 0 0 0 0 0 0 0 0]
  Constant22 : Constant  Value=[0 0 0 0 0 0 0 0 0 0 0 0 0 0 0 0 0 0 0 0 1 0 0 0 0 0 0 0 0 0 0 0 0 0 0 0 0 0 0 0 0 0 0 0 0 0 0 0 0 0 0 0 0 0 0 0 0 0 0 0 0 0 0 0]
  Constant23 : Constant  Value=[0 0 0 0 0 0 0 0 0 0 0 0 0 0 0 0 0 0 0 0 0 1 0 0 0 0 0 0 0 0 0 0 0 0 0 0 0 0 0 0 0 0 0 0 0 0 0 0 0 0 0 0 0 0 0 0 0 0 0 0 0 0 0 0]
  Constant24 : Constant  Value=[0 0 0 0 0 0 0 0 0 0 0 0 0 0 0 0 0 0 0 0 0 0 1 0 0 0 0 0 0 0 0 0 0 0 0 0 0 0 0 0 0 0 0 0 0 0 0 0 0 0 0 0 0 0 0 0 0 0 0 0 0 0 0 0]
  Constant25 : Constant  Value=[0 0 0 0 0 0 0 0 0 0 0 0 0 0 0 0 0 0 0 0 0 0 0 1 0 0 0 0 0 0 0 0 0 0 0 0 0 0 0 0 0 0 0 0 0 0 0 0 0 0 0 0 0 0 0 0 0 0 0 0 0 0 0 0]
  Constant26 : Constant  Value=[0 0 0 0 0 0 0 0 0 0 0 0 0 0 0 0 0 0 0 0 0 0 0 0 1 0 0 0 0 0 0 0 0 0 0 0 0 0 0 0 0 0 0 0 0 0 0 0 0 0 0 0 0 0 0 0 0 0 0 0 0 0 0 0]
  Constant27 : Constant  Value=[0 0 0 0 0 0 0 0 0 0 0 0 0 0 0 0 0 0 0 0 0 0 0 0 0 1 0 0 0 0 0 0 0 0 0 0 0 0 0 0 0 0 0 0 0 0 0 0 0 0 0 0 0 0 0 0 0 0 0 0 0 0 0 0]
  Constant28 : Constant  Value=[0 0 0 0 0 0 0 0 0 0 0 0 0 0 0 0 0 0 0 0 0 0 0 0 0 0 1 0 0 0 0 0 0 0 0 0 0 0 0 0 0 0 0 0 0 0 0 0 0 0 0 0 0 0 0 0 0 0 0 0 0 0 0 0]
  Constant29 : Constant  Value=[0 0 0 0 0 0 0 0 0 0 0 0 0 0 0 0 0 0 0 0 0 0 0 0 0 0 0 1 0 0 0 0 0 0 0 0 0 0 0 0 0 0 0 0 0 0 0 0 0 0 0 0 0 0 0 0 0 0 0 0 0 0 0 0]
  Constant3 : Constant  Value=[0 0 0 1 0 0 0 0 0 0 0 0 0 0 0 0 0 0 0 0 0 0 0 0 0 0 0 0 0 0 0 0 0 0 0 0 0 0 0 0 0 0 0 0 0 0 0 0 0 0 0 0 0 0 0 0 0 0 0 0 0 0 0 0]
  Constant30 : Constant  Value=[0 0 0 0 0 0 0 0 0 0 0 0 0 0 0 0 0 0 0 0 0 0 0 0 0 0 0 0 1 0 0 0 0 0 0 0 0 0 0 0 0 0 0 0 0 0 0 0 0 0 0 0 0 0 0 0 0 0 0 0 0 0 0 0]
  Constant31 : Constant  Value=[0 0 0 0 0 0 0 0 0 0 0 0 0 0 0 0 0 0 0 0 0 0 0 0 0 0 0 0 0 1 0 0 0 0 0 0 0 0 0 0 0 0 0 0 0 0 0 0 0 0 0 0 0 0 0 0 0 0 0 0 0 0 0 0]
  Constant32 : Constant  Value=[0 0 0 0 0 0 0 0 0 0 0 0 0 0 0 0 0 0 0 0 0 0 0 0 0 0 0 0 0 0 1 0 0 0 0 0 0 0 0 0 0 0 0 0 0 0 0 0 0 0 0 0 0 0 0 0 0 0 0 0 0 0 0 0]
  Constant33 : Constant  Value=[0 0 0 0 0 0 0 0 0 0 0 0 0 0 0 0 0 0 0 0 0 0 0 0 0 0 0 0 0 0 0 1 0 0 0 0 0 0 0 0 0 0 0 0 0 0 0 0 0 0 0 0 0 0 0 0 0 0 0 0 0 0 0 0]
  Constant34 : Constant  Value=[0 0 0 0 0 0 0 0 0 0 0 0 0 0 0 0 0 0 0 0 0 0 0 0 0 0 0 0 0 0 0 0 1 0 0 0 0 0 0 0 0 0 0 0 0 0 0 0 0 0 0 0 0 0 0 0 0 0 0 0 0 0 0 0]
  Constant35 : Constant  Value=[0 0 0 0 0 0 0 0 0 0 0 0 0 0 0 0 0 0 0 0 0 0 0 0 0 0 0 0 0 0 0 0 0 1 0 0 0 0 0 0 0 0 0 0 0 0 0 0 0 0 0 0 0 0 0 0 0 0 0 0 0 0 0 0]
  Constant36 : Constant  Value=[0 0 0 0 0 0 0 0 0 0 0 0 0 0 0 0 0 0 0 0 0 0 0 0 0 0 0 0 0 0 0 0 0 0 1 0 0 0 0 0 0 0 0 0 0 0 0 0 0 0 0 0 0 0 0 0 0 0 0 0 0 0 0 0]
  Constant37 : Constant  Value=[0 0 0 0 0 0 0 0 0 0 0 0 0 0 0 0 0 0 0 0 0 0 0 0 0 0 0 0 0 0 0 0 0 0 0 1 0 0 0 0 0 0 0 0 0 0 0 0 0 0 0 0 0 0 0 0 0 0 0 0 0 0 0 0]
  Constant38 : Constant  Value=[0 0 0 0 0 0 0 0 0 0 0 0 0 0 0 0 0 0 0 0 0 0 0 0 0 0 0 0 0 0 0 0 0 0 0 0 1 0 0 0 0 0 0 0 0 0 0 0 0 0 0 0 0 0 0 0 0 0 0 0 0 0 0 0]
  Constant39 : Constant  Value=[0 0 0 0 0 0 0 0 0 0 0 0 0 0 0 0 0 0 0 0 0 0 0 0 0 0 0 0 0 0 0 0 0 0 0 0 0 1 0 0 0 0 0 0 0 0 0 0 0 0 0 0 0 0 0 0 0 0 0 0 0 0 0 0]
  Constant4 : Constant  Value=[1 0 0 0 0 0 0 0 0 0 0 0 0 0 0 0 0 0 0 0 0 0 0 0 0 0 0 0 0 0 0 0 0 0 0 0 0 0 0 0 0 0 0 0 0 0 0 0 0 0 0 0 0 0 0 0 0 0 0 0 0 0 0 0]
  Constant40 : Constant  Value=[0 0 0 0 0 0 0 0 0 0 0 0 0 0 0 0 0 0 0 0 0 0 0 0 0 0 0 0 0 0 0 0 0 0 0 0 0 0 1 0 0 0 0 0 0 0 0 0 0 0 0 0 0 0 0 0 0 0 0 0 0 0 0 0]
  Constant41 : Constant  Value=[0 0 0 0 0 0 0 0 0 0 0 0 0 0 0 0 0 0 0 0 0 0 0 0 0 0 0 0 0 0 0 0 0 0 0 0 0 0 0 1 0 0 0 0 0 0 0 0 0 0 0 0 0 0 0 0 0 0 0 0 0 0 0 0]
  Constant42 : Constant  Value=[0 0 0 0 0 0 0 0 0 0 0 0 0 0 0 0 0 0 0 0 0 0 0 0 0 0 0 0 0 0 0 0 0 0 0 0 0 0 0 0 1 0 0 0 0 0 0 0 0 0 0 0 0 0 0 0 0 0 0 0 0 0 0 0]
  Constant43 : Constant  Value=[0 0 0 0 0 0 0 0 0 0 0 0 0 0 0 0 0 0 0 0 0 0 0 0 0 0 0 0 0 0 0 0 0 0 0 0 0 0 0 0 0 1 0 0 0 0 0 0 0 0 0 0 0 0 0 0 0 0 0 0 0 0 0 0]
  Constant44 : Constant  Value=[0 0 0 0 0 0 0 0 0 0 0 0 0 0 0 0 0 0 0 0 0 0 0 0 0 0 0 0 0 0 0 0 0 0 0 0 0 0 0 0 0 0 1 0 0 0 0 0 0 0 0 0 0 0 0 0 0 0 0 0 0 0 0 0]
  Constant45 : Constant  Value=[0 0 0 0 0 0 0 0 0 0 0 0 0 0 0 0 0 0 0 0 0 0 0 0 0 0 0 0 0 0 0 0 0 0 0 0 0 0 0 0 0 0 0 0 1 0 0 0 0 0 0 0 0 0 0 0 0 0 0 0 0 0 0 0]
  Constant46 : Constant  Value=[0 0 0 0 0 0 0 0 0 0 0 0 0 0 0 0 0 0 0 0 0 0 0 0 0 0 0 0 0 0 0 0 0 0 0 0 0 0 0 0 0 0 0 0 0 1 0 0 0 0 0 0 0 0 0 0 0 0 0 0 0 0 0 0]
  Constant47 : Constant  Value=[0 0 0 0 0 0 0 0 0 0 0 0 0 0 0 0 0 0 0 0 0 0 0 0 0 0 0 0 0 0 0 0 0 0 0 0 0 0 0 0 0 0 0 0 0 0 1 0 0 0 0 0 0 0 0 0 0 0 0 0 0 0 0 0]
  Constant48 : Constant  Value=[0 0 0 0 0 0 0 0 0 0 0 0 0 0 0 0 0 0 0 0 0 0 0 0 0 0 0 0 0 0 0 0 0 0 0 0 0 0 0 0 0 0 0 0 0 0 0 1 0 0 0 0 0 0 0 0 0 0 0 0 0 0 0 0]
  Constant49 : Constant  Value=[0 0 0 0 0 0 0 0 0 0 0 0 0 0 0 0 0 0 0 0 0 0 0 0 0 0 0 0 0 0 0 0 0 0 0 0 0 0 0 0 0 0 0 0 0 0 0 0 1 0 0 0 0 0 0 0 0 0 0 0 0 0 0 0]
  Constant5 : Constant  Value=[0 0 0 0 1 0 0 0 0 0 0 0 0 0 0 0 0 0 0 0 0 0 0 0 0 0 0 0 0 0 0 0 0 0 0 0 0 0 0 0 0 0 0 0 0 0 0 0 0 0 0 0 0 0 0 0 0 0 0 0 0 0 0 0]
  Constant50 : Constant  Value=[0 0 0 0 0 0 0 0 0 0 0 0 0 0 0 0 0 0 0 0 0 0 0 0 0 0 0 0 0 0 0 0 0 0 0 0 0 0 0 0 0 0 0 0 0 0 0 0 0 1 0 0 0 0 0 0 0 0 0 0 0 0 0 0]
  Constant51 : Constant  Value=[0 0 0 0 0 0 0 0 0 0 0 0 0 0 0 0 0 0 0 0 0 0 0 0 0 0 0 0 0 0 0 0 0 0 0 0 0 0 0 0 0 0 0 0 0 0 0 0 0 0 1 0 0 0 0 0 0 0 0 0 0 0 0 0]
  Constant52 : Constant  Value=[0 0 0 0 0 0 0 0 0 0 0 0 0 0 0 0 0 0 0 0 0 0 0 0 0 0 0 0 0 0 0 0 0 0 0 0 0 0 0 0 0 0 0 0 0 0 0 0 0 0 0 1 0 0 0 0 0 0 0 0 0 0 0 0]
  Constant53 : Constant  Value=[0 0 0 0 0 0 0 0 0 0 0 0 0 0 0 0 0 0 0 0 0 0 0 0 0 0 0 0 0 0 0 0 0 0 0 0 0 0 0 0 0 0 0 0 0 0 0 0 0 0 0 0 1 0 0 0 0 0 0 0 0 0 0 0]
  Constant54 : Constant  Value=[0 0 0 0 0 0 0 0 0 0 0 0 0 0 0 0 0 0 0 0 0 0 0 0 0 0 0 0 0 0 0 0 0 0 0 0 0 0 0 0 0 0 0 0 0 0 0 0 0 0 0 0 0 1 0 0 0 0 0 0 0 0 0 0]
  Constant55 : Constant  Value=[0 0 0 0 0 0 0 0 0 0 0 0 0 0 0 0 0 0 0 0 0 0 0 0 0 0 0 0 0 0 0 0 0 0 0 0 0 0 0 0 0 0 0 0 0 0 0 0 0 0 0 0 0 0 1 0 0 0 0 0 0 0 0 0]
  Constant56 : Constant  Value=[0 0 0 0 0 0 0 0 0 0 0 0 0 0 0 0 0 0 0 0 0 0 0 0 0 0 0 0 0 0 0 0 0 0 0 0 0 0 0 0 0 0 0 0 0 0 0 0 0 0 0 0 0 0 0 1 0 0 0 0 0 0 0 0]
  Constant57 : Constant  Value=[0 0 0 0 0 0 0 0 0 0 0 0 0 0 0 0 0 0 0 0 0 0 0 0 0 0 0 0 0 0 0 0 0 0 0 0 0 0 0 0 0 0 0 0 0 0 0 0 0 0 0 0 0 0 0 0 1 0 0 0 0 0 0 0]
  Constant58 : Constant  Value=[0 0 0 0 0 0 0 0 0 0 0 0 0 0 0 0 0 0 0 0 0 0 0 0 0 0 0 0 0 0 0 0 0 0 0 0 0 0 0 0 0 0 0 0 0 0 0 0 0 0 0 0 0 0 0 0 0 1 0 0 0 0 0 0]
  Constant59 : Constant  Value=[0 0 0 0 0 0 0 0 0 0 0 0 0 0 0 0 0 0 0 0 0 0 0 0 0 0 0 0 0 0 0 0 0 0 0 0 0 0 0 0 0 0 0 0 0 0 0 0 0 0 0 0 0 0 0 0 0 0 1 0 0 0 0 0]
  Constant6 : Constant  Value=[0 0 0 0 0 1 0 0 0 0 0 0 0 0 0 0 0 0 0 0 0 0 0 0 0 0 0 0 0 0 0 0 0 0 0 0 0 0 0 0 0 0 0 0 0 0 0 0 0 0 0 0 0 0 0 0 0 0 0 0 0 0 0 0]
  Constant60 : Constant  Value=[0 0 0 0 0 0 0 0 0 0 0 0 0 0 0 0 0 0 0 0 0 0 0 0 0 0 0 0 0 0 0 0 0 0 0 0 0 0 0 0 0 0 0 0 0 0 0 0 0 0 0 0 0 0 0 0 0 0 0 1 0 0 0 0]
  Constant61 : Constant  Value=[0 0 0 0 0 0 0 0 0 0 0 0 0 0 0 0 0 0 0 0 0 0 0 0 0 0 0 0 0 0 0 0 0 0 0 0 0 0 0 0 0 0 0 0 0 0 0 0 0 0 0 0 0 0 0 0 0 0 0 0 1 0 0 0]
  Constant62 : Constant  Value=[0 0 0 0 0 0 0 0 0 0 0 0 0 0 0 0 0 0 0 0 0 0 0 0 0 0 0 0 0 0 0 0 0 0 0 0 0 0 0 0 0 0 0 0 0 0 0 0 0 0 0 0 0 0 0 0 0 0 0 0 0 1 0 0]
  Constant63 : Constant  Value=[0 0 0 0 0 0 0 0 0 0 0 0 0 0 0 0 0 0 0 0 0 0 0 0 0 0 0 0 0 0 0 0 0 0 0 0 0 0 0 0 0 0 0 0 0 0 0 0 0 0 0 0 0 0 0 0 0 0 0 0 0 0 1 0]
  Constant64 : Constant  Value=[0 0 0 0 0 0 0 0 0 0 0 0 0 0 0 0 0 0 0 0 0 0 0 0 0 0 0 0 0 0 0 0 0 0 0 0 0 0 0 0 0 0 0 0 0 0 0 0 0 0 0 0 0 0 0 0 0 0 0 0 0 0 0 1]
  Constant7 : Constant  Value=[0 0 0 0 0 0 1 0 0 0 0 0 0 0 0 0 0 0 0 0 0 0 0 0 0 0 0 0 0 0 0 0 0 0 0 0 0 0 0 0 0 0 0 0 0 0 0 0 0 0 0 0 0 0 0 0 0 0 0 0 0 0 0 0]
  Constant8 : Constant  Value=[0 0 0 0 0 0 0 1 0 0 0 0 0 0 0 0 0 0 0 0 0 0 0 0 0 0 0 0 0 0 0 0 0 0 0 0 0 0 0 0 0 0 0 0 0 0 0 0 0 0 0 0 0 0 0 0 0 0 0 0 0 0 0 0]
  Constant9 : Constant  Value=[0 0 0 0 0 0 0 0 1 0 0 0 0 0 0 0 0 0 0 0 0 0 0 0 0 0 0 0 0 0 0 0 0 0 0 0 0 0 0 0 0 0 0 0 0 0 0 0 0 0 0 0 0 0 0 0 0 0 0 0 0 0 0 0]
  Data_1 : Subsystem  mask{a=0}
  Data_10 : Subsystem  mask{a=9}
  Data_11 : Subsystem  mask{a=10}
  Data_12 : Subsystem  mask{a=11}
  Data_13 : Subsystem  mask{a=12}
  Data_14 : Subsystem  mask{a=13}
  Data_15 : Subsystem  mask{a=14}
  Data_16 : Subsystem  mask{a=15}
  Data_17 : Subsystem  mask{a=16}
  Data_18 : Subsystem  mask{a=17}
  Data_19 : Subsystem  mask{a=18}
  Data_2 : Subsystem  mask{a=1}
  Data_20 : Subsystem  mask{a=19}
  Data_21 : Subsystem  mask{a=20}
  Data_22 : Subsystem  mask{a=21}
  Data_23 : Subsystem  mask{a=22}
  Data_24 : Subsystem  mask{a=23}
  Data_25 : Subsystem  mask{a=24}
  Data_26 : Subsystem  mask{a=25}
  Data_27 : Subsystem  mask{a=26}
  Data_28 : Subsystem  mask{a=27}
  Data_29 : Subsystem  mask{a=28}
  Data_3 : Subsystem  mask{a=2}
  Data_30 : Subsystem  mask{a=29}
  Data_31 : Subsystem  mask{a=30}
  Data_32 : Subsystem  mask{a=31}
  Data_33 : Subsystem  mask{a=32}
  Data_34 : Subsystem  mask{a=33}
  Data_35 : Subsystem  mask{a=34}
  Data_36 : Subsystem  mask{a=35}
  Data_37 : Subsystem  mask{a=36}
  Data_38 : Subsystem  mask{a=37}
  Data_39 : Subsystem  mask{a=38}
  Data_4 : Subsystem  mask{a=3}
  Data_40 : Subsystem  mask{a=39}
  Data_41 : Subsystem  mask{a=40}
  Data_42 : Subsystem  mask{a=41}
  Data_43 : Subsystem  mask{a=42}
  Data_44 : Subsystem  mask{a=43}
  Data_45 : Subsystem  mask{a=44}
  Data_46 : Subsystem  mask{a=45}
  Data_47 : Subsystem  mask{a=46}
  Data_48 : Subsystem  mask{a=47}
  Data_49 : Subsystem  mask{a=48}
  Data_5 : Subsystem  mask{a=4}
  Data_50 : Subsystem  mask{a=49}
  Data_51 : Subsystem  mask{a=50}
  Data_52 : Subsystem  mask{a=51}
  Data_53 : Subsystem  mask{a=52}
  Data_54 : Subsystem  mask{a=53}
  Data_55 : Subsystem  mask{a=54}
  Data_56 : Subsystem  mask{a=55}
  Data_57 : Subsystem  mask{a=56}
  Data_58 : Subsystem  mask{a=57}
  Data_59 : Subsystem  mask{a=58}
  Data_6 : Subsystem  mask{a=5}
  Data_60 : Subsystem  mask{a=59}
  Data_61 : Subsystem  mask{a=60}
  Data_62 : Subsystem  mask{a=61}
  Data_63 : Subsystem  mask{a=62}
  Data_64 : Subsystem  mask{a=63}
  Data_7 : Subsystem  mask{a=6}
  Data_8 : Subsystem  mask{a=7}
  Data_9 : Subsystem  mask{a=8}
  Divide{,1..63} (64 alike) : Product  Inputs=**  Multiplication=Matrix(*)
  Math Function{,1..64} (65 alike) : Math  Operator=transpose  SaturateOnIntegerOverflow=on
  Rate Transition : RateTransition  Deterministic=off
  Rate Transition3 : RateTransition  Deterministic=off
  Rate Transition5 : RateTransition  Deterministic=off
  ESR_Data[64X4] : Outport
  tag scope: ESRcal=global
  wires:
  Constant4/1 -> Math Function/1
  Math Function/1 -> Divide/2
  Divide/1 -> Add/1
  Constant1/1 -> Math Function1/1
  Math Function1/1 -> Divide1/2
  Divide1/1 -> Add/2
  Constant2/1 -> Math Function2/1
  Math Function2/1 -> Divide2/2
  Divide2/1 -> Add/3
  Constant3/1 -> Math Function3/1
  Math Function3/1 -> Divide3/2
  Divide3/1 -> Add/4
  Constant5/1 -> Math Function4/1
  Math Function4/1 -> Divide4/2
  Divide4/1 -> Add/5
  Constant6/1 -> Math Function5/1
  Math Function5/1 -> Divide5/2
  Divide5/1 -> Add/6
  Constant7/1 -> Math Function6/1
  Math Function6/1 -> Divide6/2
  Divide6/1 -> Add/7
  Constant8/1 -> Math Function7/1
  Math Function7/1 -> Divide7/2
  Divide7/1 -> Add/8
  Constant9/1 -> Math Function8/1
  Math Function8/1 -> Divide8/2
  Divide8/1 -> Add/9
  Constant10/1 -> Math Function9/1
  Math Function9/1 -> Divide9/2
  Divide9/1 -> Add/10
  Constant11/1 -> Math Function10/1
  Math Function10/1 -> Divide10/2
  Divide10/1 -> Add/11
  Constant12/1 -> Math Function11/1
  Math Function11/1 -> Divide11/2
  Divide11/1 -> Add/12
  Constant13/1 -> Math Function12/1
  Math Function12/1 -> Divide12/2
  Divide12/1 -> Add/13
  Constant14/1 -> Math Function13/1
  Math Function13/1 -> Divide13/2
  Divide13/1 -> Add/14
  Constant16/1 -> Math Function14/1
  Math Function14/1 -> Divide14/2
  Divide14/1 -> Add/15
  Constant17/1 -> Math Function15/1
  Math Function15/1 -> Divide15/2
  Divide15/1 -> Add/16
  Constant18/1 -> Math Function16/1
  Math Function16/1 -> Divide16/2
  Divide16/1 -> Add/17
  Constant19/1 -> Math Function17/1
  Math Function17/1 -> Divide17/2
  Divide17/1 -> Add/18
  Constant20/1 -> Math Function18/1
  Math Function18/1 -> Divide18/2
  Divide18/1 -> Add/19
  Constant21/1 -> Math Function19/1
  Math Function19/1 -> Divide19/2
  Divide19/1 -> Add/20
  Constant22/1 -> Math Function20/1
  Math Function20/1 -> Divide20/2
  Divide20/1 -> Add/21
  Constant23/1 -> Math Function21/1
  Math Function21/1 -> Divide21/2
  Divide21/1 -> Add/22
  Constant24/1 -> Math Function22/1
  Math Function22/1 -> Divide22/2
  Divide22/1 -> Add/23
  Constant25/1 -> Math Function23/1
  Math Function23/1 -> Divide23/2
  Divide23/1 -> Add/24
  Constant26/1 -> Math Function24/1
  Math Function24/1 -> Divide24/2
  Divide24/1 -> Add/25
  Constant27/1 -> Math Function25/1
  Math Function25/1 -> Divide25/2
  Divide25/1 -> Add/26
  Constant28/1 -> Math Function26/1
  Math Function26/1 -> Divide26/2
  Divide26/1 -> Add/27
  Constant29/1 -> Math Function27/1
  Math Function27/1 -> Divide27/2
  Divide27/1 -> Add/28
  Constant30/1 -> Math Function28/1
  Math Function28/1 -> Divide28/2
  Divide28/1 -> Add/29
  Constant31/1 -> Math Function29/1
  Math Function29/1 -> Divide29/2
  Divide29/1 -> Add/30
  Constant32/1 -> Math Function30/1
  Math Function30/1 -> Divide30/2
  Divide30/1 -> Add/31
  Constant33/1 -> Math Function31/1
  Math Function31/1 -> Divide31/2
  Divide31/1 -> Add/32
  Constant34/1 -> Math Function32/1
  Math Function32/1 -> Divide32/2
  Divide32/1 -> Add/33
  Constant35/1 -> Math Function33/1
  Math Function33/1 -> Divide33/2
  Divide33/1 -> Add/34
  Constant36/1 -> Math Function34/1
  Math Function34/1 -> Divide34/2
  Divide34/1 -> Add/35
  Constant37/1 -> Math Function35/1
  Math Function35/1 -> Divide35/2
  Divide35/1 -> Add/36
  Constant38/1 -> Math Function36/1
  Math Function36/1 -> Divide36/2
  Divide36/1 -> Add/37
  Constant39/1 -> Math Function37/1
  Math Function37/1 -> Divide37/2
  Divide37/1 -> Add/38
  Constant40/1 -> Math Function38/1
  Divide38/1 -> Add/39
  Math Function38/1 -> Divide38/2
  Math Function45/1 -> Divide45/2
  Constant49/1 -> Math Function48/1
  Constant46/1 -> Math Function45/1
  Divide49/1 -> Add/50
  Divide45/1 -> Add/46
  Math Function48/1 -> Divide48/2
  Math Function49/1 -> Divide49/2
  Constant50/1 -> Math Function49/1
  Divide48/1 -> Add/49
  Constant41/1 -> Math Function39/1
  Math Function39/1 -> Divide39/2
  Divide39/1 -> Add/40
  Math Function40/1 -> Divide40/2
  Divide40/1 -> Add/41
  Constant42/1 -> Math Function40/1
  Constant43/1 -> Math Function41/1
  Divide41/1 -> Add/42
  Math Function41/1 -> Divide41/2
  Divide42/1 -> Add/43
  Math Function42/1 -> Divide42/2
  Constant44/1 -> Math Function42/1
  Math Function43/1 -> Divide43/2
  Divide43/1 -> Add/44
  Constant15/1 -> Math Function43/1
  Divide46/1 -> Add/47
  Math Function46/1 -> Divide46/2
  Constant47/1 -> Math Function46/1
  Constant48/1 -> Math Function47/1
  Math Function47/1 -> Divide47/2
  Divide47/1 -> Add/48
  Constant45/1 -> Math Function44/1
  Math Function44/1 -> Divide44/2
  Divide44/1 -> Add/45
  Constant54/1 -> Math Function53/1
  Math Function53/1 -> Divide53/2
  Divide53/1 -> Add/54
  Math Function54/1 -> Divide54/2
  Constant55/1 -> Math Function54/1
  Divide54/1 -> Add/55
  Math Function50/1 -> Divide50/2
  Divide50/1 -> Add/51
  Constant51/1 -> Math Function50/1
  Divide51/1 -> Add/52
  Math Function51/1 -> Divide51/2
  Constant52/1 -> Math Function51/1
  Constant56/1 -> Math Function55/1
  Math Function55/1 -> Divide55/2
  Divide55/1 -> Add/56
  Divide57/1 -> Add/58
  Math Function57/1 -> Divide57/2
  Constant58/1 -> Math Function57/1
  Constant53/1 -> Math Function52/1
  Math Function52/1 -> Divide52/2
  Divide52/1 -> Add/53
  Divide59/1 -> Add/60
  Constant60/1 -> Math Function59/1
  Math Function59/1 -> Divide59/2
  Divide56/1 -> Add/57
  Math Function56/1 -> Divide56/2
  Constant57/1 -> Math Function56/1
  Divide58/1 -> Add/59
  Math Function58/1 -> Divide58/2
  Constant59/1 -> Math Function58/1
  Divide60/1 -> Add/61
  Math Function60/1 -> Divide60/2
  Constant61/1 -> Math Function60/1
  Constant63/1 -> Math Function62/1
  Math Function62/1 -> Divide62/2
  Divide62/1 -> Add/63
  Constant62/1 -> Math Function61/1
  Math Function61/1 -> Divide61/2
  Divide61/1 -> Add/62
  Math Function63/1 -> Divide63/2
  Divide63/1 -> Add/64
  Constant64/1 -> Math Function63/1
  Add/1 -> Math Function64/1
  Math Function64/1 -> Rate Transition/1
  Chart/1(DataOutput) -> Rate Transition3/1
  Rate Transition/1 -> Chart/1(DataInput)
  Chart2/1(count) -> Rate Transition5/1
  Rate Transition5/1 -> Chart/Trigger, [ESRcal]
  CAN_TYPE1_INT_M1_C1_ESR/1 -> Chart2/Trigger
  Rate Transition3/1 -> ESR_Data[64X4]/1
  Data_1/1(Out1) -> Divide/1
  Data_2/1(Out1) -> Divide1/1
  Data_3/1(Out1) -> Divide2/1
  Data_4/1(Out1) -> Divide3/1
  Data_5/1(Out1) -> Divide4/1
  Data_6/1(Out1) -> Divide5/1
  Data_7/1(Out1) -> Divide6/1
  Data_8/1(Out1) -> Divide7/1
  Data_9/1(Out1) -> Divide8/1
  Data_10/1(Out1) -> Divide9/1
  Data_11/1(Out1) -> Divide10/1
  Data_12/1(Out1) -> Divide11/1
  Data_13/1(Out1) -> Divide12/1
  Data_14/1(Out1) -> Divide13/1
  Data_15/1(Out1) -> Divide14/1
  Data_16/1(Out1) -> Divide15/1
  Data_17/1(Out1) -> Divide16/1
  Data_18/1(Out1) -> Divide17/1
  Data_19/1(Out1) -> Divide18/1
  Data_20/1(Out1) -> Divide19/1
  Data_21/1(Out1) -> Divide20/1
  Data_22/1(Out1) -> Divide21/1
  Data_23/1(Out1) -> Divide22/1
  Data_24/1(Out1) -> Divide23/1
  Data_25/1(Out1) -> Divide24/1
  Data_26/1(Out1) -> Divide25/1
  Data_27/1(Out1) -> Divide26/1
  Data_28/1(Out1) -> Divide27/1
  Data_29/1(Out1) -> Divide28/1
  Data_30/1(Out1) -> Divide29/1
  Data_31/1(Out1) -> Divide30/1
  Data_32/1(Out1) -> Divide31/1
  Data_33/1(Out1) -> Divide32/1
  Data_34/1(Out1) -> Divide33/1
  Data_35/1(Out1) -> Divide34/1
  Data_36/1(Out1) -> Divide35/1
  Data_37/1(Out1) -> Divide36/1
  Data_38/1(Out1) -> Divide37/1
  Data_39/1(Out1) -> Divide38/1
  Data_40/1(Out1) -> Divide39/1
  Data_41/1(Out1) -> Divide40/1
  Data_42/1(Out1) -> Divide41/1
  Data_43/1(Out1) -> Divide42/1
  Data_44/1(Out1) -> Divide43/1
  Data_45/1(Out1) -> Divide44/1
  Data_46/1(Out1) -> Divide45/1
  Data_47/1(Out1) -> Divide46/1
  Data_48/1(Out1) -> Divide47/1
  Data_49/1(Out1) -> Divide48/1
  Data_50/1(Out1) -> Divide49/1
  Data_51/1(Out1) -> Divide50/1
  Data_52/1(Out1) -> Divide51/1
  Data_53/1(Out1) -> Divide52/1
  Data_54/1(Out1) -> Divide53/1
  Data_55/1(Out1) -> Divide54/1
  Data_56/1(Out1) -> Divide55/1
  Data_57/1(Out1) -> Divide56/1
  Data_58/1(Out1) -> Divide57/1
  Data_59/1(Out1) -> Divide58/1
  Data_60/1(Out1) -> Divide59/1
  Data_61/1(Out1) -> Divide60/1
  Data_62/1(Out1) -> Divide61/1
  Data_63/1(Out1) -> Divide62/1
  Data_64/1(Out1) -> Divide63/1

== system ADU_Integration_Y2016_simulation/LogData/Vision_Target ==
  note: This part is used for ensure the sensor data is from once update
  1-D Lookup Table : Lookup_n-D  NumberOfTableDimensions=1  BreakpointsForDimension1=TestData_001.X.Data  Table=TestData_001.Y(662).Data  RndMeth=Simplest  InputSameDT=on
  CameraData : Subsystem
  Chart1 : Stateflow chart  TreatAsAtomicUnit=on
  EPM_Lane_Signals : Subsystem
  Vision_Target[25x8] : Outport
  EPM_Lane : Outport  Port=2
  tag scope: CameraCal=global, CameraTime=global
  wires:
  EPM_Lane_Signals/1(EPM_Lane_Singals) -> EPM_Lane/1
  [Clock] -> Chart1/2(Time), 1-D Lookup Table/1
  Chart1/1(Time_out) -> [CameraTime]
  1-D Lookup Table/1 -> [CameraCal], Chart1/1(Trig)
  Chart1/2(DataOutput) -> Vision_Target[25x8]/1
  CameraData/1(CameraData[25X8]) -> Chart1/3(DataInput)
